simulink model "speedController"  (R2016b)
settings: Solver=FixedStepAuto  StartTime=0.0  StopTime=inf  RelTol=1e-3
undefined symbols (not defined in the file): Angular, Linear
libraries: robotlib x12
settings Model: Creator=jupan  LastModifiedBy=jupan
settings OptimizationCC: MaxStackSize=64
settings DebuggingCC: ParameterTunabilityLossMsg=error
settings HardwareCC: ProdBitPerPointer=32  ProdBitPerSizeT=32  ProdBitPerPtrDiffT=32  ProdLargestAtomicFloat=None  ProdIntDivRoundTo=Undefined  ProdEndianess=Unspecified  ProdWordSize=32  ProdHWDeviceType=Generic->Unspecified (assume 32-bit Generic)
settings RTWCC: SystemTargetFile=ert.tlc  HardwareBoard=Robot Operating System (ROS)  TLCOptions="-aInlineSetEventsForThisBaseRateFcn=TLC_FALSE -aSuppressMultiTaskScheduler=TLC_FALSE  -aRateBasedStepFcn=0"  TemplateMakefile=ert_default_tmf  Description=Embedded Coder  GenerateReport=on  Toolchain=Catkin  IncludeHyperlinkInReport=on  LaunchReport=on  TargetLang=C++  GenerateTraceInfo=on  GenerateTraceReport=on  GenerateTraceReportSl=on  GenerateTraceReportSf=on  GenerateTraceReportEml=on
settings CodeAppCC: ForceParamTrailComments=on  IgnoreCustomStorageClasses=off  OperatorAnnotations=on  SimulinkDataObjDesc=on  SFDataObjDesc=on  MATLABFcnDesc=on  InsertBlockDesc=on  MATLABSourceComments=on

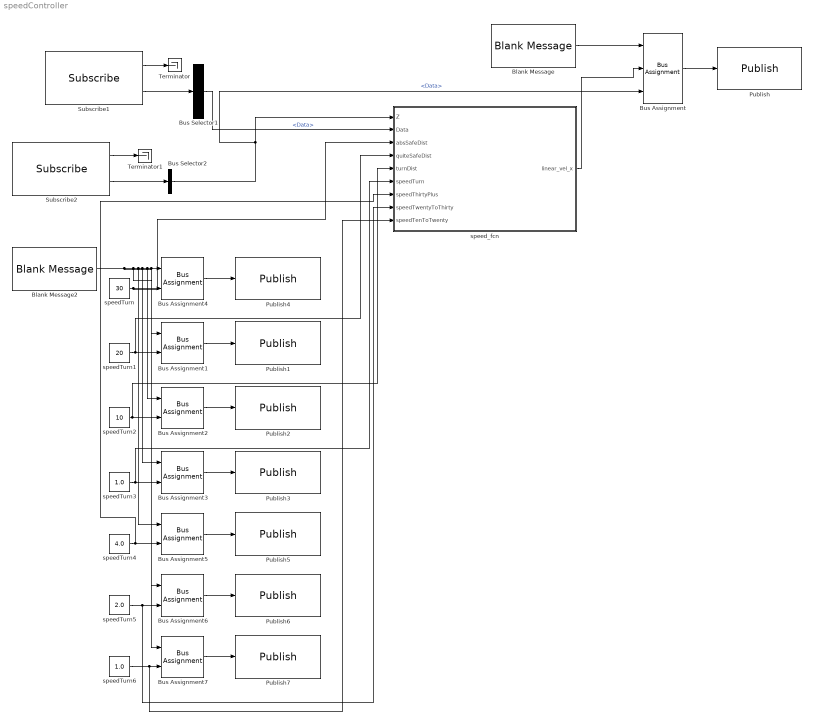
== system speedController ==
  Blank Message : robotlib/Blank Message  SourceLibraryInfo=This block requires Robotics System Toolbox  messageType=geometry_msgs/Twist  SampleTime=inf
  Blank Message2 : robotlib/Blank Message  SourceLibraryInfo=This block requires Robotics System Toolbox  messageType=std_msgs/Float64  SampleTime=1.0
  Bus Assignment : BusAssignment  AssignedSignals=Linear.X,Angular.Z
  Bus Assignment{1..7} (7 alike) : BusAssignment  AssignedSignals=Data
  Bus Selector1 : BusSelector  OutputSignals=Data
  Bus Selector2 : BusSelector  OutputSignals=Data
  Publish : robotlib/Publish  SourceLibraryInfo=This block requires Robotics System Toolbox  topicSource=Select from ROS network  topic=/catvehicle/cmd_vel  messageType=geometry_msgs/Twist  messageQueueLength=1
  Publish1 : robotlib/Publish  SourceLibraryInfo=This block requires Robotics System Toolbox  topicSource=Specify your own  topic=/quiteSafeDist  messageType=std_msgs/Float64  messageQueueLength=1
  Publish2 : robotlib/Publish  SourceLibraryInfo=This block requires Robotics System Toolbox  topicSource=Specify your own  topic=/turnDist  messageType=std_msgs/Float64  messageQueueLength=1
  Publish3 : robotlib/Publish  SourceLibraryInfo=This block requires Robotics System Toolbox  topicSource=Specify your own  topic=/speedTurn  messageType=std_msgs/Float64  messageQueueLength=1
  Publish4 : robotlib/Publish  SourceLibraryInfo=This block requires Robotics System Toolbox  topicSource=Specify your own  topic=/absSafeDist  messageType=std_msgs/Float64  messageQueueLength=1
  Publish5 : robotlib/Publish  SourceLibraryInfo=This block requires Robotics System Toolbox  topicSource=Specify your own  topic=/speedThirtyPlus  messageType=std_msgs/Float64  messageQueueLength=1
  Publish6 : robotlib/Publish  SourceLibraryInfo=This block requires Robotics System Toolbox  topicSource=Specify your own  topic=/speedTwentyToThirty  messageType=std_msgs/Float64  messageQueueLength=1
  Publish7 : robotlib/Publish  SourceLibraryInfo=This block requires Robotics System Toolbox  topicSource=Specify your own  topic=/speedTenToTwenty  messageType=std_msgs/Float64  messageQueueLength=1
  Subscribe1 : robotlib/Subscribe  SourceLibraryInfo=This block requires Robotics System Toolbox  topicSource=Select from ROS network  topic=/catvehicle/distanceEstimator/dist  messageType=std_msgs/Float32  sampleTime=-1  messageQueueLength=1
  Subscribe2 : robotlib/Subscribe  SourceLibraryInfo=This block requires Robotics System Toolbox  topicSource=Specify your own  topic=/direction  messageType=std_msgs/Float64  sampleTime=-1  messageQueueLength=1
  Terminator : Terminator
  Terminator1 : Terminator
  speedTurn : Constant  Value=30  OutDataTypeStr=double
  speedTurn1 : Constant  Value=20  OutDataTypeStr=double
  speedTurn2 : Constant  Value=10  OutDataTypeStr=double
  speedTurn3 : Constant  Value=1.0  OutDataTypeStr=double
  speedTurn4 : Constant  Value=4.0  OutDataTypeStr=double
  speedTurn5 : Constant  Value=2.0  OutDataTypeStr=double
  speedTurn6 : Constant  Value=1.0  OutDataTypeStr=double
  speed_fcn : MATLAB Function  TreatAsAtomicUnit=on
  wires:
  Blank Message/1 -> Bus Assignment/1
  Bus Assignment/1 -> Publish/1
  speed_fcn/1(linear_vel_x) -> Bus Assignment/2
  Subscribe2/2 -> Bus Selector2/1
  Bus Selector2/1 -> Bus Assignment/3, speed_fcn/1(Z)  "<Data>"
  Subscribe2/1 -> Terminator1/1
  Subscribe1/2 -> Bus Selector1/1
  Subscribe1/1 -> Terminator/1
  Bus Selector1/1 -> speed_fcn/2(Data)  "<Data>"
  Bus Assignment4/1 -> Publish4/1
  Blank Message2/1 -> Bus Assignment7/1, Bus Assignment6/1, Bus Assignment5/1, Bus Assignment3/1, Bus Assignment2/1, Bus Assignment1/1, Bus Assignment4/1
  Bus Assignment1/1 -> Publish1/1
  Bus Assignment2/1 -> Publish2/1
  Bus Assignment3/1 -> Publish3/1
  Bus Assignment5/1 -> Publish5/1
  Bus Assignment6/1 -> Publish6/1
  Bus Assignment7/1 -> Publish7/1
  speedTurn/1 -> speed_fcn/3(absSafeDist), Bus Assignment4/2
  speedTurn1/1 -> speed_fcn/4(quiteSafeDist), Bus Assignment1/2
  speedTurn2/1 -> speed_fcn/5(turnDist), Bus Assignment2/2
  speedTurn3/1 -> speed_fcn/6(speedTurn), Bus Assignment3/2
  speedTurn4/1 -> speed_fcn/7(speedThirtyPlus), Bus Assignment5/2
  speedTurn5/1 -> speed_fcn/8(speedTwentyToThirty), Bus Assignment6/2
  speedTurn6/1 -> speed_fcn/9(speedTenToTwenty), Bus Assignment7/2

== matlab function speedController/speed_fcn ==
  data: Z input; Data input; absSafeDist input; quiteSafeDist input; turnDist input; linear_vel_x output; speedTurn input; speedThirtyPlus input; speedTwentyToThirty input; speedTenToTwenty input
function linear_vel_x = fcn(Z, Data,absSafeDist,quiteSafeDist,turnDist...
    ,speedTurn,speedThirtyPlus,speedTwentyToThirty,speedTenToTwenty)
if(Z ~= 0)
    linear_vel_x = speedTurn;
else
    if(Data >= absSafeDist)
        linear_vel_x = speedThirtyPlus;
    elseif(Data >= quiteSafeDist && Data < absSafeDist)
        linear_vel_x = speedTwentyToThirty;
    elseif(Data >= turnDist && Data < quiteSafeDist)
        linear_vel_x = speedTenToTwenty;
    else
        linear_vel_x = speedThirtyPlus;
    end
end
